simulink model "MS_alimentation_IS_autopilotage"  (Simulink 7.8)
settings: Solver=ode45  StartTime=0.0  StopTime=0.050  MaxStep=100e-6  RelTol=1e-6
undefined symbols (not defined in the file): Ts
libraries: powerlib x18, powerlib_extras x3
settings Model: Creator=obethoux  LastModifiedBy=obethoux

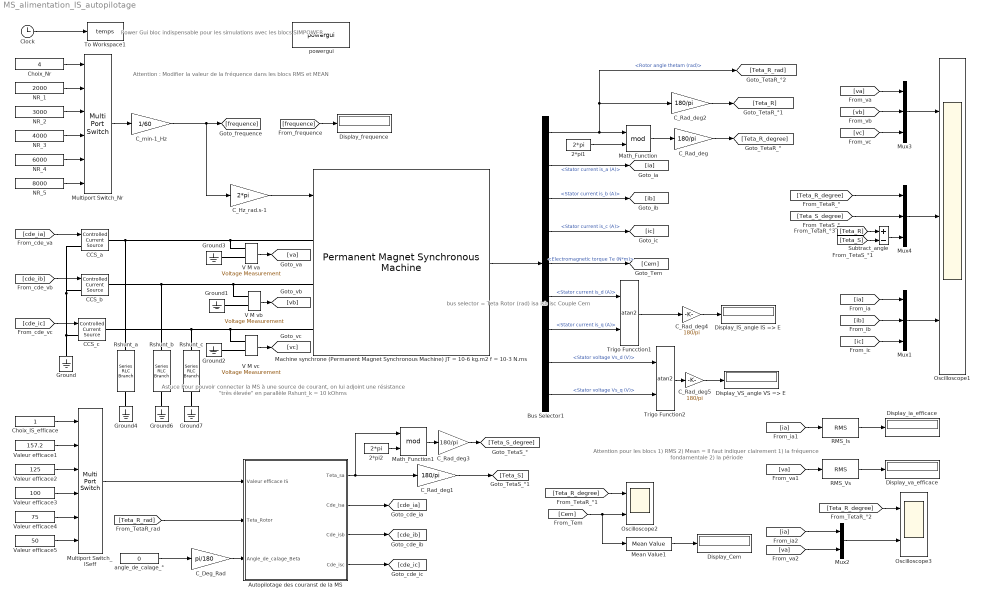
== system MS_alimentation_IS_autopilotage ==
  note: Power Gui
      | bloc indispensable pour les simulations
      | avec les blocs SIMPOWER
  note: bus selector
      | =
      | Teta Rotor (rad)
      | isa
      | isb
      | isc
      | Couple Cem
  note: Attention pour les blocs
      | 1) RMS
      | 2) Mean
      | =
      | Il faut indiquer clairement
      | 1) la fréquence fondamentale
      | 2) la période
  note: Astuce
      | Pour pouvoir connecter la MS à une source de courant,
      | on lui adjoint une résistance "très élevée" en parallèle
      | Rshunt_k = 10 kOhms
  note: Attention : Modifier la valeur de la fréquence dans les blocs RMS et MEAN
  2*pi1 : Constant  Value=2*pi
  2*pi2 : Constant  Value=2*pi
  Autopilotage des couranst de la MS : Subsystem
  Bus Selector1 : BusSelector  OutputSignals=Rotor angle thetam (rad),Stator current is_a (A),Stator current is_b (A),Stator current is_c (A),Electromagnetic torque Te (N*m),Stator current is_d (A),Stator current is_q (A),Stator voltage Vs_d (V),Stator voltage Vs_q (V)
  CCS_a : powerlib/Electrical Sources/Controlled Current Source  Initialize=on  Source_Type=AC  Amplitude=0  Phase=0  Frequency=0  Measurements=None
  CCS_b : powerlib/Electrical Sources/Controlled Current Source  Initialize=on  Source_Type=AC  Amplitude=0  Phase=0  Frequency=0  Measurements=None
  CCS_c : powerlib/Electrical Sources/Controlled Current Source  Initialize=on  Source_Type=AC  Amplitude=0  Phase=0  Frequency=0  Measurements=None
  C_Deg_Rad : Gain  Gain=pi/180
  C_Hz_rad.s-1 : Gain  Gain=2*pi
  C_Rad_deg{,1..5} (6 alike) : Gain  Gain=180/pi
  C_min-1_Hz : Gain  Gain=1/60
  Choix_IS_efficace : Constant
  Choix_Nr : Constant  Value=4
  Clock : Clock
  Display_Cem : Display
      settings: Decimation=100
  Display_IS_angle IS => E : Display
      settings: Decimation=100
  Display_VS_angle VS => E : Display
      settings: Decimation=100
  Display_frequence : Display
      settings: Decimation=1000
  Display_ia_efficace : Display
      settings: Decimation=100
  Display_va_efficace : Display
      settings: Decimation=100
  Ground{,1..4,6..7} (7 alike) : powerlib/Elements/Ground  LConnTagsString=a
  "Machine synchrone (Permanent Magnet Synchronous Machine) JT = 10-6 kg.m2 f = 10-3 N.ms " : powerlib/Machines/Permanent Magnet Synchronous Machine  NbPhases=3  FluxDistribution=Sinusoidal  RotorType=Round  MechanicalLoad=Speed w  PresetModel=No  ShowDetailedParameters=on  Resistance=6.75e-3  Inductance=8.5e-3  dqInductances=[8.5e-3,8.5e-3]  La=1.61e-3  MachineConstant=Flux linkage established by magnets (V.s)  Flux=358.1e-3  VoltageCst=64.9522  TorqueCst=0.53715  Flat=120  Mechanical=[1e-6 1e-3 1 0]  PolePairs=1  InitialConditions=[0,0, 0,0]  InitialConditions5ph=[0 0 0 0 0 0]  TsPowergui=0  TsBlock=-1  RefAngle=90 degrees behind phase A axis (modified Park)
  Math_Function : Math  Operator=mod  SaturateOnIntegerOverflow=on
  Math_Function1 : Math  Operator=mod  SaturateOnIntegerOverflow=on
  Mean Value1 : powerlib_extras/Measurements/Mean Value  Period=inv(100)
  Multiport Switch_ISeff : MultiPortSwitch  Inputs=5  zeroidx=off
  Multiport Switch_Nr : MultiPortSwitch  Inputs=5  zeroidx=off
  Mux1 : Mux  Inputs=3
  Mux2 : Mux  Inputs=2
  Mux3 : Mux  Inputs=3
  Mux4 : Mux  Inputs=3
  NR_1 : Constant  Value=2000
  NR_2 : Constant  Value=3000
  NR_3 : Constant  Value=4000
  NR_4 : Constant  Value=6000
  NR_5 : Constant  Value=8000
  Oscilloscope1 : Scope  NumInputPorts=3
      settings: YMin=-125~0~-250  YMax=150~400~250  SaveName=ScopeData2
  Oscilloscope2 : Scope  NumInputPorts=2
      settings: YMin=0~-125  YMax=375~125
  Oscilloscope3 : Scope  NumInputPorts=2
      settings: YMin=0~-225  YMax=225~150
  RMS_Is : powerlib_extras/Measurements/RMS  f1=100
  RMS_Vs : powerlib_extras/Measurements/RMS  f1=100
  Rshunt_a : powerlib/Elements/Series RLC Branch  LConnTagsString=__new0  RConnTagsString=__new0  BranchType=R  Resistance=1e4  Inductance=1e-3  SetiL0=off  InitialCurrent=0  Capacitance=1e-6  Setx0=off  InitialVoltage=0  Measurements=Branch voltage
  Rshunt_b : powerlib/Elements/Series RLC Branch  LConnTagsString=__new0  RConnTagsString=__new0  BranchType=R  Resistance=1e4  Inductance=1e-3  SetiL0=off  InitialCurrent=0  Capacitance=1e-6  Setx0=off  InitialVoltage=0  Measurements=Branch voltage
  Rshunt_c : powerlib/Elements/Series RLC Branch  LConnTagsString=__new0  RConnTagsString=__new0  BranchType=R  Resistance=1e4  Inductance=1e-3  SetiL0=off  InitialCurrent=0  Capacitance=1e-6  Setx0=off  InitialVoltage=0  Measurements=Branch voltage
  Subtract_angle : Sum  Inputs=+-
  To Workspace1 : ToWorkspace  VariableName=temps  SampleTime=-1  SaveFormat=Array
  Trigo Funcction1 : Trigonometry  Operator=atan2
  Trigo Function2 : Trigonometry  Operator=atan2
  V M va : powerlib/Measurements/Voltage Measurement  PhasorSimulation=off  OutputType=Complex  PSBequivalent=0
  V M vb : powerlib/Measurements/Voltage Measurement  PhasorSimulation=off  OutputType=Complex  PSBequivalent=0
  V M vc : powerlib/Measurements/Voltage Measurement  PhasorSimulation=off  OutputType=Complex  PSBequivalent=0
  Valeur efficace1 : Constant  Value=157.2
  Valeur efficace2 : Constant  Value=125
  Valeur efficace3 : Constant  Value=100
  Valeur efficace4 : Constant  Value=75
  Valeur efficace5 : Constant  Value=50
  angle_de_calage_° : Constant  Value=0
  powergui : powerlib/powergui  Priority=2  SimulationMode=Continuous  SolverType=Tustin  SampleTime=Ts  frequency=60  SPID=off  DisableSnubberDevices=off  DisableRonSwitches=off  DisableVfSwitches=off  SwTol=0  Interpol=off  DisplayEquations=off  FunctionMessages=off  frequencyindice=0  Pbase=100e6  ErrMax=1e-4  Iterations=50  UnitsV=kV  UnitsW=MW  echomessages=off  HookPort=off  EnableUseOfTLC=off  x0status=blocks  RestoreLinks=warning  ResistiveCurrentMeasurement=off  Frange=[0:2:500]  Ylog=off  Xlog=on  ShowGrid=off  save=off  variable=ZData  ZoomFFT=on  StartTime=0.0  cycles=1  DisplayStyle=1  fundamental=60  FreqAxis=off  MaxFrequency=1000  frequencyindicesteady=1  RmsSteady=1  display=off  Ts=0  methode=off
  wires:
  Clock/1 -> To Workspace1/1
  "Machine synchrone (Permanent Magnet Synchronous Machine) JT = 10-6 kg.m2 f = 10-3 N.ms "/1 -> Bus Selector1/1
  Mux3/1 -> Oscilloscope1/1
  [ia] -> Mux1/1
  [ib] -> Mux1/2
  [ic] -> Mux1/3
  [va] -> Mux3/1
  [vb] -> Mux3/2
  [vc] -> Mux3/3
  [Teta_R_rad] -> Autopilotage des couranst de la MS/2(Teta_Rotor)
  Autopilotage des couranst de la MS/2(Cde_isa) -> [cde_ia]
  Autopilotage des couranst de la MS/3(Cde_isb) -> [cde_ib]
  Autopilotage des couranst de la MS/4(Cde_isc) -> [cde_ic]
  [cde_ia] -> CCS_a/1
  [cde_ic] -> CCS_c/1
  [cde_ib] -> CCS_b/1
  Mux1/1 -> Oscilloscope1/3
  [ia] -> RMS_Is/1
  RMS_Is/1 -> Display_ia_efficace/1
  [va] -> RMS_Vs/1
  RMS_Vs/1 -> Display_va_efficace/1
  [Teta_R_degree] -> Oscilloscope2/1
  [Cem] -> Oscilloscope2/2, Mean Value1/1
  Mean Value1/1 -> Display_Cem/1
  V M va/1 -> [va]
  V M vb/1 -> [vb]
  V M vc/1 -> [vc]
  Valeur efficace1/1 -> Multiport Switch_ISeff/2
  Multiport Switch_ISeff/1 -> Autopilotage des couranst de la MS/1(Valeur efficace IS)
  Valeur efficace2/1 -> Multiport Switch_ISeff/3
  Valeur efficace3/1 -> Multiport Switch_ISeff/4
  Choix_IS_efficace/1 -> Multiport Switch_ISeff/1
  Valeur efficace4/1 -> Multiport Switch_ISeff/5
  Valeur efficace5/1 -> Multiport Switch_ISeff/6
  Mux2/1 -> Oscilloscope3/2
  [Teta_R_degree] -> Oscilloscope3/1
  [va] -> Mux2/2
  [ia] -> Mux2/1
  Multiport Switch_Nr/1 -> C_min-1_Hz/1
  NR_1/1 -> Multiport Switch_Nr/2
  Choix_Nr/1 -> Multiport Switch_Nr/1
  angle_de_calage_°/1 -> C_Deg_Rad/1
  NR_2/1 -> Multiport Switch_Nr/3
  NR_3/1 -> Multiport Switch_Nr/4
  NR_4/1 -> Multiport Switch_Nr/5
  NR_5/1 -> Multiport Switch_Nr/6
  C_min-1_Hz/1 -> C_Hz_rad.s-1/1, [frequence]
  C_Hz_rad.s-1/1 -> "Machine synchrone (Permanent Magnet Synchronous Machine) JT = 10-6 kg.m2 f = 10-3 N.ms "/1
  [frequence] -> Display_frequence/1
  C_Deg_Rad/1 -> Autopilotage des couranst de la MS/3(Angle_de_calage_Beta)
  Bus Selector1/1 -> Math_Function/1, C_Rad_deg2/1, [Teta_R_rad]  "<Rotor angle thetam (rad)>"
  2*pi1/1 -> Math_Function/2
  Math_Function/1 -> C_Rad_deg/1
  Bus Selector1/2 -> [ia]  "<Stator current is_a (A)>"
  Bus Selector1/3 -> [ib]  "<Stator current is_b (A)>"
  Bus Selector1/4 -> [ic]  "<Stator current is_c (A)>"
  Bus Selector1/5 -> [Cem]  "<Electromagnetic torque Te (N*m)>"
  C_Rad_deg/1 -> [Teta_R_degree]
  C_Rad_deg2/1 -> [Teta_R]
  Trigo Funcction1/1 -> C_Rad_deg4/1
  Trigo Function2/1 -> C_Rad_deg5/1
  C_Rad_deg4/1 -> Display_IS_angle IS => E/1
  C_Rad_deg5/1 -> Display_VS_angle VS => E/1
  Bus Selector1/6 -> Trigo Funcction1/1  "<Stator current is_d (A)>"
  Bus Selector1/7 -> Trigo Funcction1/2  "<Stator current is_q (A)>"
  Bus Selector1/8 -> Trigo Function2/1  "<Stator voltage Vs_d (V)>"
  Bus Selector1/9 -> Trigo Function2/2  "<Stator voltage Vs_q (V)>"
  [Teta_R_degree] -> Mux4/1
  Subtract_angle/1 -> Mux4/3
  [Teta_S_degree] -> Mux4/2
  Mux4/1 -> Oscilloscope1/2
  [Teta_R] -> Subtract_angle/1
  [Teta_S] -> Subtract_angle/2
  2*pi2/1 -> Math_Function1/2
  Autopilotage des couranst de la MS/1(Teta_sa) -> Math_Function1/1, C_Rad_deg1/1
  C_Rad_deg1/1 -> [Teta_S]
  Math_Function1/1 -> C_Rad_deg3/1
  C_Rad_deg3/1 -> [Teta_S_degree]
  connections:
  CCS_c/LConn1 -- CCS_a/LConn1 -- CCS_b/LConn1 -- Ground/LConn1
  Ground3/LConn1 -- V M va/LConn2
  Ground1/LConn1 -- V M vb/LConn2
  V M vc/LConn2 -- Ground2/LConn1
  "Machine synchrone (Permanent Magnet Synchronous Machine) JT = 10-6 kg.m2 f = 10-3 N.ms "/LConn1 -- V M va/LConn1 -- CCS_a/RConn1 -- Rshunt_a/LConn1
  "Machine synchrone (Permanent Magnet Synchronous Machine) JT = 10-6 kg.m2 f = 10-3 N.ms "/LConn2 -- V M vb/LConn1 -- CCS_b/RConn1 -- Rshunt_b/LConn1
  "Machine synchrone (Permanent Magnet Synchronous Machine) JT = 10-6 kg.m2 f = 10-3 N.ms "/LConn3 -- V M vc/LConn1 -- CCS_c/RConn1 -- Rshunt_c/LConn1
  Ground4/LConn1 -- Rshunt_a/RConn1
  Ground6/LConn1 -- Rshunt_b/RConn1
  Ground7/LConn1 -- Rshunt_c/RConn1

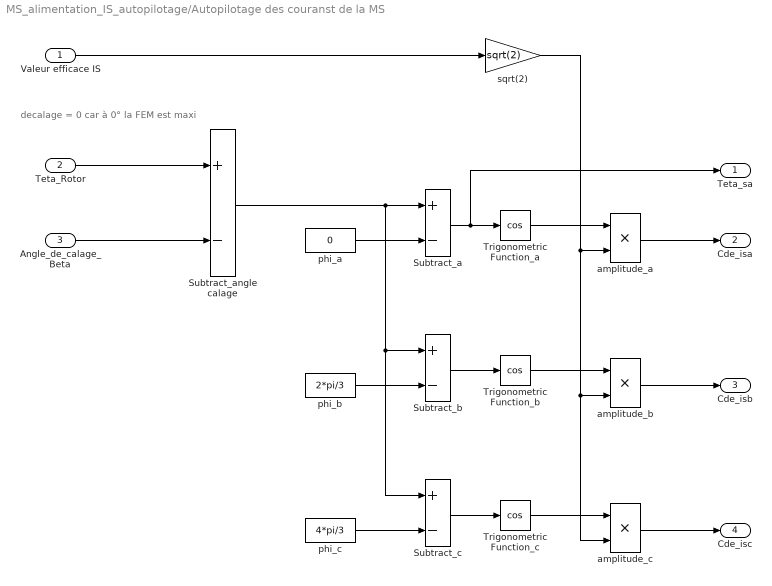
== system MS_alimentation_IS_autopilotage/Autopilotage des couranst de la MS ==
  note: decalage = 0 car à 0° la FEM est maxi
  Valeur efficace IS : Inport
  Teta_Rotor : Inport  Port=2
  Angle_de_calage_Beta : Inport  Port=3
  Subtract_a : Sum  Inputs=+-
  Subtract_angle calage : Sum  Inputs=+-
  Subtract_b : Sum  Inputs=+-
  Subtract_c : Sum  Inputs=+-
  Trigonometric Function_a : Trigonometry  Operator=cos
  Trigonometric Function_b : Trigonometry  Operator=cos
  Trigonometric Function_c : Trigonometry  Operator=cos
  amplitude_a : Product  RndMeth=Zero
  amplitude_b : Product  RndMeth=Zero
  amplitude_c : Product  RndMeth=Zero
  phi_a : Constant  Value=0
  phi_b : Constant  Value=2*pi/3
  phi_c : Constant  Value=4*pi/3
  sqrt(2) : Gain  Gain=sqrt(2)
  Teta_sa : Outport
  Cde_isa : Outport  Port=2
  Cde_isb : Outport  Port=3
  Cde_isc : Outport  Port=4
  wires:
  Subtract_angle calage/1 -> Subtract_a/1, Subtract_b/1, Subtract_c/1
  phi_a/1 -> Subtract_a/2
  phi_b/1 -> Subtract_b/2
  phi_c/1 -> Subtract_c/2
  Subtract_a/1 -> Trigonometric Function_a/1, Teta_sa/1
  Subtract_b/1 -> Trigonometric Function_b/1
  Subtract_c/1 -> Trigonometric Function_c/1
  Trigonometric Function_a/1 -> amplitude_a/1
  Trigonometric Function_b/1 -> amplitude_b/1
  Trigonometric Function_c/1 -> amplitude_c/1
  sqrt(2)/1 -> amplitude_a/2, amplitude_b/2, amplitude_c/2
  Valeur efficace IS/1 -> sqrt(2)/1
  amplitude_a/1 -> Cde_isa/1
  amplitude_b/1 -> Cde_isb/1
  amplitude_c/1 -> Cde_isc/1
  Angle_de_calage_Beta/1 -> Subtract_angle calage/2
  Teta_Rotor/1 -> Subtract_angle calage/1
